simulink model "Lab4"  (Simulink 3.00)
settings: Solver=ode45  SolverMode=SingleTasking  StartTime=0.0  StopTime=10.0  RelTol=1e-3  AbsTol=1e-6
undefined symbols (not defined in the file): sfunyst
settings Model: RTWTemplateMakefile=grt_unix.tmf  Creator=vise  LastModifiedBy=vise

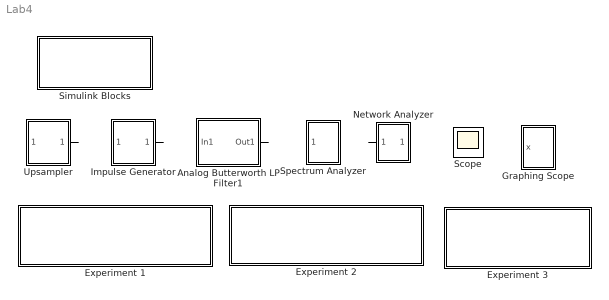
== system Lab4 ==
  Analog Butterworth LP Filter1 : Subsystem  mask(buttap){@1=2*pi, @2=10}
      mask prompts: @1 "Cutoff frequency (rad/sec)"; @2 "Order"
      mask help:
      | Analog Butterworth low pass filter.
      |
      | (Requires Signal Processing Toolbox)
      mask init:
      | [z,p,k]=buttap(@2); z=@1*z; p=@1*p; k=real(prod(-p)); [num,den]=zp2tf(z,p,k); w=logspace(log10(@1/10),log10(10*@1),20); h=freqs(num,den,w);
      mask Help: Butterworth low pass filter using MATLAB's butter command.
      mask Display: plot(20*log10(w),20*log10(abs(h)))
  Experiment 1 : Subsystem
      settings: OpenFcn=ImpulseGen
      mask Type: Impulse Generator
      mask Display: disp('Sampling and Reconstruction \n Using an Inpulse Generator')
  Experiment 2 : Subsystem
      settings: OpenFcn=SampHold
      mask Type: Sample and Hold
      mask Display: disp('Sampling and Reconstruction \nUsing a Sample and Hold')
  Experiment 3 : Subsystem  Orientation=left
      settings: OpenFcn=Interp
      mask Type: Interpolator
      mask Display: disp('Discrete Time \nInterpolator')
  Graphing Scope : Subsystem  mask(Storage scope.){@1=20, @2=-1.5, @3=1.5, @4=500, @5='r-/b--/g-./w:/m*/ro/b+'}
      mask prompts: @1 "Initial Time Range:"; @2 "Initial y-min:"; @3 "Initial y-max:"; @4 "Storage pts.:"; @5 "Line type (rgbw-.:xo):"
      mask help:
      | Storage scope using MATLAB graph window.
      | Enter plotting ranges and line type.
      mask init:
      | npts = @4; color = @5; ax = [0, @1, @2, @3]; dt=-1;
      mask Help: This block uses a MATLAB figure window to plot the input signal.  The graph limits are automatically scaled to the min and max values of the signal stored in the scope's signal buffer.  Line type must be in quotes.  See the M-file sfunyst.m.
      mask Display: plot(0,0,100,100,[83,76,63,52,42,38,28,16,11,84,11,11,11,90,90,11],[75,58,47,54,72,80,84,74,65,65,65,90,40,40,90,90])
  Impulse Generator : Subsystem  mask(D-T interpolator){@1=1, @2=0.2}
      mask prompts: @1 "Input sampling period:"; @2 "Pulse width:"
      mask init:
      | T=@1;L=round(@1/@2);
      mask Display: plot(-10,-10,110,110,[0,50,50,60,60,100],[0,0,80,80,0,0])
  Network Analyzer : Subsystem  Orientation=left  mask(Network Analyzer){@1=256, @2=0.1}
      mask prompts: @1 "Number of sample points:"; @2 "Sampling period (sec):"
      mask init:
      | max_freq=0.9*pi/@2;N=@1;T_s=@2;const=2*pi/(@1*@2);window1=0.5*@1*@2;window2=@1*@2;
      mask Help: Estimates frequency response of system using chirp input. Used for EE438. See Prof. Bouman.
      mask Display: plot(0,0,100,100,[11,93,93,11,11],[90,90,40,40,90],[80,60,40,20],[50,79,50,80])
  Scope : Scope
      settings: TickLabels=on  TimeRange=auto  YMin=-5  YMax=5  SaveToWorkspace=off  SaveName=ScopeData  DataFormat=Matrix
  Simulink Blocks : Subsystem
      settings: OpenFcn=simulink
      mask Type: Waveform Synthesizer
      mask Display: disp('Full Block Library')
  Spectrum Analyzer : Subsystem  mask(Spectrum analyzer.){@1=2048, @2=0.02, @3=10}
      mask prompts: @1 "Number of sample points:"; @2 "Sampling period (sec):"; @3 "Plotting Period (sec):"
      mask init:
      | N=@1; T_s=@2;plot_period=@3;
      mask Help: EE438 Lab utility; See Prof. Bouman.
      mask Display: plot(0,0,100,100,[14,91,91,14,14],[86,86,40,40,86],[85,82,80,79,75,67,63,60,57,53,41,36,33,27,24],[49,50,53,50,49,51,54,66,54,50,50,52,81,51,49])
  Upsampler : Subsystem  mask(D-T interpolator){@1=1, @2=1}
      mask prompts: @1 "Input sampling period:"; @2 "Upsampling factor:"
      mask init:
      | T=@1;L=@2;
      mask Display: disp('L')
  wires:
  ? -> Analog Butterworth LP Filter1/1(In1)
  Analog Butterworth LP Filter1/1(Out1) -> ?
  ? -> Impulse Generator/1(in_1)
  Impulse Generator/1(out_1) -> ?
  ? -> Network Analyzer/1(Inport)
  Network Analyzer/1(Outport) -> ?
  ? -> Spectrum Analyzer/1(input signal)
  ? -> Upsampler/1(in_1)
  Upsampler/1(out_1) -> ?

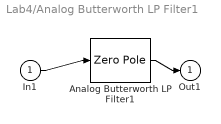
== system Lab4/Analog Butterworth LP Filter1 ==
  In1 : Inport  Port=1  PortWidth=-1  SampleTime=-1  DataType=auto
      settings: SignalType=auto
  Analog Butterworth LP Filter1 : ZeroPole  Zeros=z  Poles=p  Gain=k
  Out1 : Outport  Port=1
  wires:
  In1/1 -> Analog Butterworth LP Filter1/1
  Analog Butterworth LP Filter1/1 -> Out1/1

== system Lab4/Experiment 1 ==

== system Lab4/Experiment 2 ==

== system Lab4/Experiment 3 ==

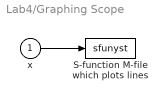
== system Lab4/Graphing Scope ==
  x : Inport  Port=1  PortWidth=-1  SampleTime=-1  DataType=auto
      settings: SignalType=auto
  "S-function M-file which plots lines " : S-Function  LoadFcn=sfunyst([],[],[],'LoadBlock')  FunctionName=sfunyst  Parameters=ax, color, npts, dt  PortCounts=[]  SFunctionModules=''
      settings: CopyFcn=sfunyst([],[],[],'CopyBlock')  DeleteFcn=sfunyst([],[],[],'DeleteBlock')
  wires:
  x/1 -> "S-function M-file which plots lines "/1

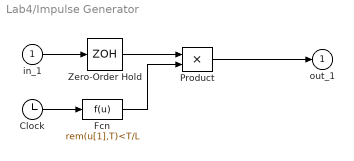
== system Lab4/Impulse Generator ==
  in_1 : Inport  Port=1  PortWidth=-1  SampleTime=-1  DataType=auto
      settings: SignalType=auto
  Clock : Clock
      settings: DisplayTime=off  Decimation=10
  Fcn : Fcn  Expr=rem(u[1],T)<T/L
  Product : Product  Inputs=2  SaturateOnIntegerOverflow=on
  Zero-Order Hold : ZeroOrderHold  SampleTime=T
  out_1 : Outport  Port=1  InitialOutput=0
  wires:
  in_1/1 -> Zero-Order Hold/1
  Zero-Order Hold/1 -> Product/1
  Fcn/1 -> Product/2
  Product/1 -> out_1/1
  Clock/1 -> Fcn/1

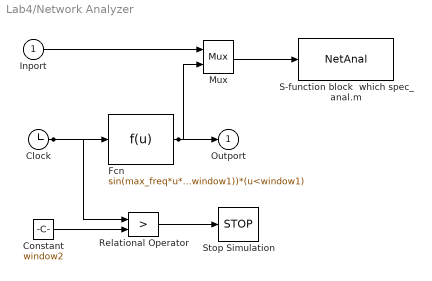
== system Lab4/Network Analyzer ==
  Inport : Inport  Port=1  PortWidth=-1  SampleTime=-1  DataType=auto
      settings: SignalType=auto
  Clock : Clock
      settings: DisplayTime=off  Decimation=10
  Constant : Constant  Value=window2
  Fcn : Fcn  Expr=sin(max_freq*u*u/(2*window1))*(0.54+0.46*cos(pi*u/window1))*(u<window1)
  Mux : Mux  Inputs=2
      settings: DisplayOption=none
  Relational Operator : RelationalOperator  Operator=>
  S-function block  which spec_anal.m : S-Function  FunctionName=NetAnal  Parameters=N,T_s  PortCounts=[]  SFunctionModules=''
  Stop Simulation : Stop
  Outport : Outport  Port=1  InitialOutput=0
  wires:
  Inport/1 -> Mux/1
  Fcn/1 -> Mux/2, Outport/1
  Mux/1 -> S-function block  which spec_anal.m/1
  Clock/1 -> Fcn/1, Relational Operator/1
  Constant/1 -> Relational Operator/2
  Relational Operator/1 -> Stop Simulation/1

== system Lab4/Simulink Blocks ==

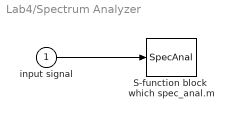
== system Lab4/Spectrum Analyzer ==
  input signal : Inport  Port=1  PortWidth=-1  SampleTime=-1  DataType=auto
      settings: SignalType=auto
  S-function block  which spec_anal.m : S-Function  FunctionName=SpecAnal  Parameters=N,T_s,plot_period  PortCounts=[]  SFunctionModules=''
  wires:
  input signal/1 -> S-function block  which spec_anal.m/1

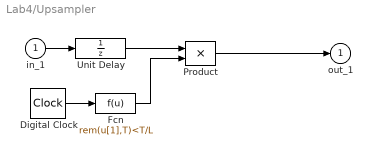
== system Lab4/Upsampler ==
  in_1 : Inport  Port=1  PortWidth=-1  SampleTime=-1  DataType=auto
      settings: SignalType=auto
  Digital Clock : DigitalClock  SampleTime=T/L
  Fcn : Fcn  Expr=rem(u[1],T)<T/L
  Product : Product  Inputs=2  SaturateOnIntegerOverflow=on
  Unit Delay : UnitDelay  X0=0  SampleTime=T/L
  out_1 : Outport  Port=1  InitialOutput=0
  wires:
  Product/1 -> out_1/1
  Fcn/1 -> Product/2
  Unit Delay/1 -> Product/1
  in_1/1 -> Unit Delay/1
  Digital Clock/1 -> Fcn/1
